simulink model "sist_cont_dt"  (Simulink 7.2)
settings: Solver=ode45  StartTime=0.0  StopTime=10.0  RelTol=1e-3
libraries: simulink_extras x1
settings Model: Creator=crisgc  LastModifiedBy=CrisGC

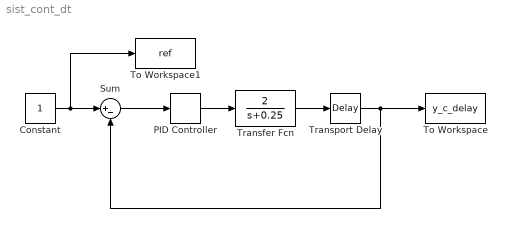
== system sist_cont_dt ==
  Constant : Constant  OutDataType=sfix(16)  OutScaling=2^0
  PID Controller : simulink_extras/Additional Linear/PID Controller  SystemSampleTime=-1  P=1  I=0.2  D=0
  Sum : Sum  Inputs=|+-  OutDataType=sfix(16)  OutScaling=2^0
  To Workspace : ToWorkspace  VariableName=y_c_delay  SampleTime=-1  SaveFormat=Array
  To Workspace1 : ToWorkspace  VariableName=ref  SampleTime=-1  SaveFormat=Array
  Transfer Fcn : TransferFcn  Numerator=[2]  Denominator=[1 0.25]
  Transport Delay : TransportDelay
  wires:
  Constant/1 -> Sum/1, To Workspace1/1
  Sum/1 -> PID Controller/1
  PID Controller/1 -> Transfer Fcn/1
  Transfer Fcn/1 -> Transport Delay/1
  Transport Delay/1 -> Sum/2, To Workspace/1
